simulink model "gm_rx_dma_test"  (R2024a)
settings: Solver=FixedStepDiscrete  StartTime=0.0  StopTime=2e-3  RelTol=1e-3  EnableMultiTasking=on
PreLoadFcn:
  | ldcr_hdl_init();
InitFcn:
  | ldcr_hdl_init();
model workspace (MAT data in the model file):
  socvcb = containers.Map
  socvcb.serialization.keys = {}
  socvcb.serialization.values = {}
  socvcb.serialization.uniformity = 0
  socvcb.serialization.keyType = 'double'
  socvcb.serialization.valueType = 'any'
libraries: dspsrcs4 x2, hdlsllib x2, dsphdlfiltering2 x1
Description:
  | libiioSDRPSP_filter_example
  | 
  | A simple example model to demonstrate the use of MATLAB I/O alongside
  | hardware/software co-design.
  | 
  | Implements AXI programmable gain and bypassable filters on the Tx and Rx
  | paths of the HDL DUT.
settings Model: SimulationMode=accelerator  ExtModeTrigDuration=100  Creator=mfornero  LastModifiedBy=versal
settings SolverCC: AlgebraicLoopSolver=TrustRegion  PositivePriorityOrder=on  MaxZcPerStep=1
settings DataIOCC: SaveOutput=off  ReturnWorkspaceOutputs=off  StateSaveName=tmp_raccel_xout  SignalLoggingName=tmp_raccel_logsout
settings OptimizationCC: BlockReduction=off  ConditionallyExecuteInputs=off  DefaultParameterBehavior=Inlined  EnhancedBackFolding=on  PassReuseOutputArgsAs=Individual arguments  ZeroExternalMemoryAtStartup=off  ZeroInternalMemoryAtStartup=off  EfficientMapNaN2IntZero=off  MaxStackSize=64  OptimizeBlockOrder=speed  DifferentSizesBufferReuse=on  OptimizationCustomize=off  EfficientTunableParamExpr=on
settings DebuggingCC: AlgebraicLoopMsg=error  InheritedTsInSrcMsg=none  SingleTaskRateTransMsg=error  ParameterTunabilityLossMsg=error  UnconnectedInputMsg=warning  UnconnectedOutputMsg=warning  UnconnectedLineMsg=warning  PregeneratedLibrarySubsystemCodeDiagnostic=none  StrictBusMsg=ErrorOnBusTreatedAsVector  SFUnexpectedBacktrackingDiag=warning  SFNoUnconditionalDefaultTransitionDiag=warning  SFExecutionAtInitializationDiag=none  ArithmeticOperatorsInVariantConditions=warning
settings HardwareCC: ProdBitPerPointer=32  ProdBitPerSizeT=32  ProdBitPerPtrDiffT=32  ProdLargestAtomicFloat=None  ProdIntDivRoundTo=Undefined  ProdEndianess=Unspecified  ProdWordSize=32  ProdHWDeviceType=ASIC/FPGA->ASIC/FPGA  TargetBitPerLong=64  TargetBitPerPointer=64  TargetBitPerSizeT=64  TargetBitPerPtrDiffT=64  TargetLongLongMode=on  TargetIntDivRoundTo=Zero  TargetEndianess=LittleEndian  TargetWordSize=64  TargetHWDeviceType=Custom Processor->MATLAB Host Computer  ProdEqTarget=off  HardwareBoardFeatureSet=SoCBlockset
settings ModelReferenceCC: EnableRefExpFcnMdlSchedulingChecks=on  ModelReferenceNumInstancesAllowed=Single
settings SFSimCC: SimUseLocalCustomCode=off  CustomCodeUndefinedFunction=UseInterfaceOnly
settings RTWCC: Description=Embedded Coder  SystemTargetFile=ert.tlc  HardwareBoard=Custom Hardware Board  TLCOptions="-aInlineSetEventsForThisBaseRateFcn=TLC_FALSE -aSuppressMultiTaskScheduler=TLC_FALSE  -aRateBasedStepFcn=0"  TemplateMakefile=ert_default_tmf  RTWVerbose=off  RTWUseLocalCustomCode=off  RTWUseSimCustomCode=on  GPUComputeCapability=3.5  DLArmComputeVersion=19.05
settings CodeAppCC: ForceParamTrailComments=on  IgnoreCustomStorageClasses=off  MaxIdLength=128  OperatorAnnotations=on  SimulinkDataObjDesc=on  SFDataObjDesc=on  MangleLength=10  InsertBlockDesc=on
settings ERTTargetCC: InlinedParameterPlacement=NonHierarchical
settings ConfigComp: CovMetricSettings=dw  CovSaveCumulativeToWorkspaceVar=on  CovSaveSingleToWorkspaceVar=on  CovExternalEMLEnable=off

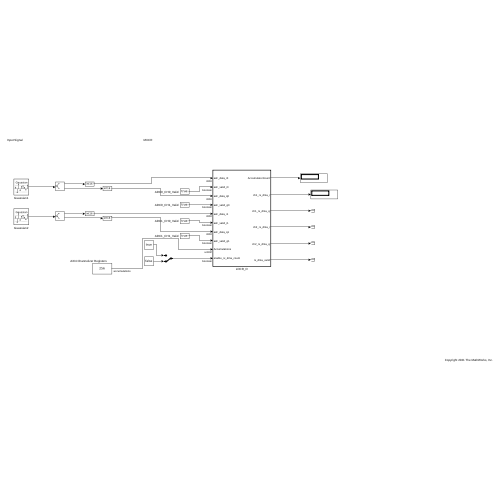
[thumbnail: Simulink's stored preview of the top-level diagram]
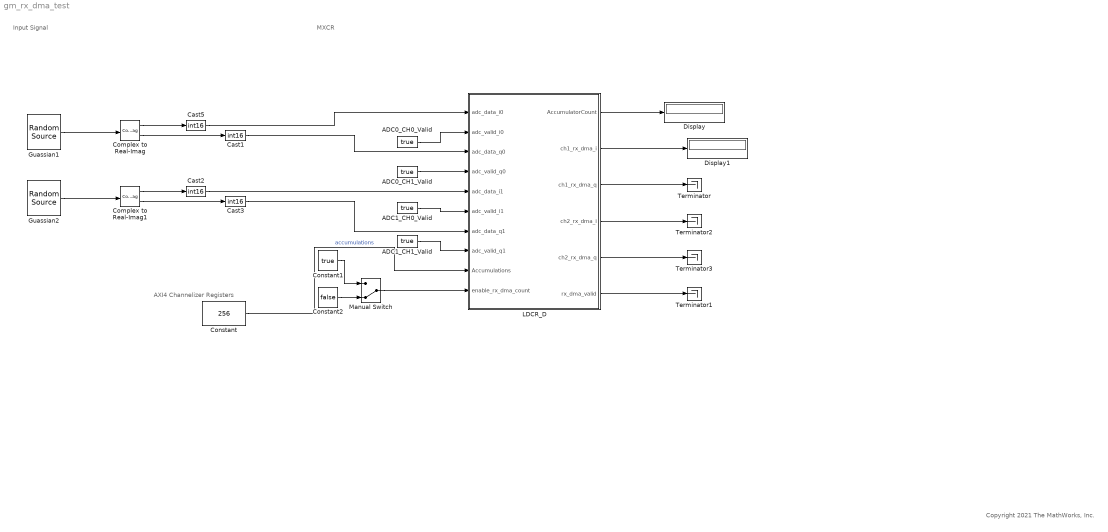
== system gm_rx_dma_test ==
  note: Input Signal
  note: MXCR
  note: Copyright 2021 The MathWorks, Inc.
  note: AXI4 Channelizer Registers
  ADC0_CH0_Valid : Constant  Value=true  SampleTime=-1
  ADC0_CH1_Valid : Constant  Value=true  SampleTime=-1
  ADC1_CH0_Valid : Constant  Value=true  SampleTime=-1
  ADC1_CH1_Valid : Constant  Value=true  SampleTime=-1
  Cast{1..3,5} (4 alike) : DataTypeConversion  OutDataTypeStr=int16  SaturateOnIntegerOverflow=off  RndMeth=Floor
  Complex to Real-Imag : ComplexToRealImag
  Complex to Real-Imag1 : ComplexToRealImag
  Constant : Constant  Value=256  OutDataTypeStr=uint32
  Constant1 : Constant  Value=true  SampleTime=-1
  Constant2 : Constant  Value=false  SampleTime=-1
  Display : Display
  Display1 : Display
  Guassian1 : dspsrcs4/Random Source  SrcType=Gaussian  MinVal=0  MaxVal=1  MeanVal=9  VarVal=24^2  RepMode=Specify seed  rawSeed=6547597  IsInherit=off  SampTime=Ts  SampFrame=1  OutComplex=Complex  DataType=single  SimulateUsing=Interpreted execution
  Guassian2 : dspsrcs4/Random Source  SrcType=Gaussian  MinVal=0  MaxVal=1  MeanVal=7  VarVal=24^2  RepMode=Specify seed  rawSeed=1324634  IsInherit=off  SampTime=Ts  SampFrame=1  OutComplex=Complex  DataType=single  SimulateUsing=Interpreted execution
  LDCR_D : Subsystem  TreatAsAtomicUnit=on
  Manual Switch : ManualSwitch  CurrentSetting=0
  Terminator{,1..3} (4 alike) : Terminator
  wires:
  Constant2/1 -> Manual Switch/2
  Constant1/1 -> Manual Switch/1
  LDCR_D/5(ch2_rx_dma_q) -> Terminator3/1
  LDCR_D/4(ch2_rx_dma_i) -> Terminator2/1
  LDCR_D/6(rx_dma_valid) -> Terminator1/1
  LDCR_D/3(ch1_rx_dma_q) -> Terminator/1
  Guassian2/1 -> Complex to Real-Imag1/1
  Guassian1/1 -> Complex to Real-Imag/1
  Cast3/1 -> LDCR_D/7(adc_data_q1)
  Cast2/1 -> LDCR_D/5(adc_data_i1)
  Cast1/1 -> LDCR_D/3(adc_data_q0)
  Cast5/1 -> LDCR_D/1(adc_data_i0)
  Complex to Real-Imag1/2 -> Cast3/1
  Complex to Real-Imag1/1 -> Cast2/1
  Complex to Real-Imag/2 -> Cast1/1
  Complex to Real-Imag/1 -> Cast5/1
  LDCR_D/1(AccumulatorCount) -> Display/1
  LDCR_D/2(ch1_rx_dma_i) -> Display1/1
  Manual Switch/1 -> LDCR_D/10(enable_rx_dma_count)
  ADC1_CH1_Valid/1 -> LDCR_D/8(adc_valid_q1)
  ADC1_CH0_Valid/1 -> LDCR_D/6(adc_valid_i1)
  ADC0_CH1_Valid/1 -> LDCR_D/4(adc_valid_q0)
  Constant/1 -> LDCR_D/9(Accumulations)  "accumulations"
  ADC0_CH0_Valid/1 -> LDCR_D/2(adc_valid_i0)

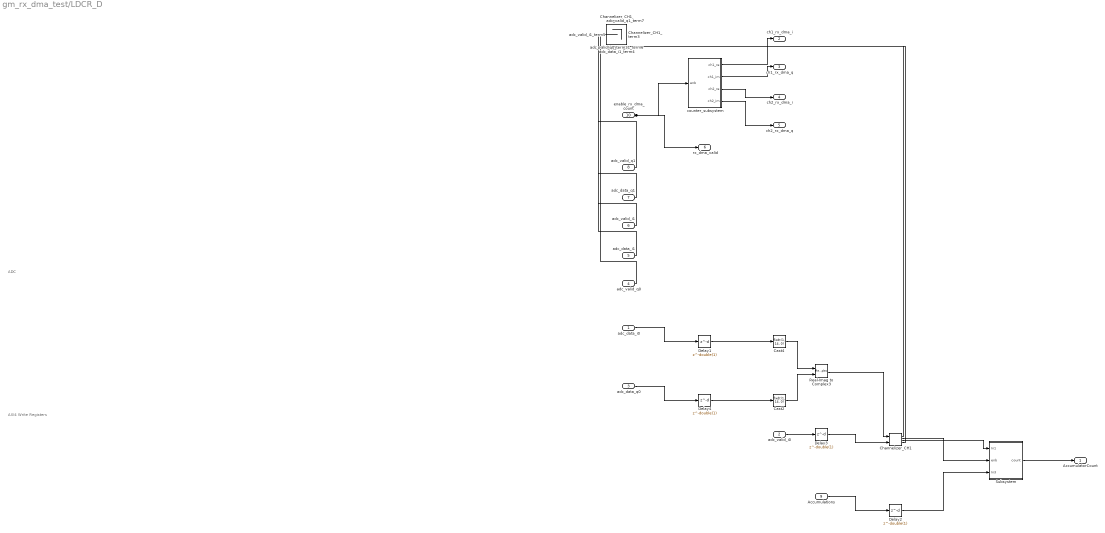
== system gm_rx_dma_test/LDCR_D ==
  note: ADC
  note: AXI4 Write Registers
  adc_data_i0 : Inport  OutDataTypeStr=int16  PortDimensions=1  SampleTime=3.25520833333333e-08
  adc_valid_i0 : Inport  Port=2  OutDataTypeStr=boolean  PortDimensions=1  SampleTime=3.25520833333333e-08
  adc_data_q0 : Inport  Port=3  OutDataTypeStr=int16  PortDimensions=1  SampleTime=3.25520833333333e-08
  adc_valid_q0 : Inport  Port=4  OutDataTypeStr=boolean  PortDimensions=1  SampleTime=3.25520833333333e-08
  adc_data_i1 : Inport  Port=5  OutDataTypeStr=int16  PortDimensions=1  SampleTime=3.25520833333333e-08
  adc_valid_i1 : Inport  Port=6  OutDataTypeStr=boolean  PortDimensions=1  SampleTime=3.25520833333333e-08
  adc_data_q1 : Inport  Port=7  OutDataTypeStr=int16  PortDimensions=1  SampleTime=3.25520833333333e-08
  adc_valid_q1 : Inport  Port=8  OutDataTypeStr=boolean  PortDimensions=1  SampleTime=3.25520833333333e-08
  Accumulations : Inport  Port=9  OutDataTypeStr=uint32  PortDimensions=1  SampleTime=3.25520833333333e-08
  enable_rx_dma_count : Inport  Port=10  OutDataTypeStr=boolean  PortDimensions=1  SampleTime=3.25520833333333e-08
  Cast2 : DataTypeConversion  OutDataTypeStr=fixdt(1, 14, 0)  SampleTime=3.25520833333333e-08  SaturateOnIntegerOverflow=off  RndMeth=Floor
  Cast4 : DataTypeConversion  OutDataTypeStr=fixdt(1, 14, 0)  SampleTime=3.25520833333333e-08  SaturateOnIntegerOverflow=off  RndMeth=Floor
  Channelizer_CH1 : dsphdlfiltering2/Channelizer  FilterCoefficients=pfb.coeffs.Numerator  FilterStructure=Direct form systolic  NumFrequencyBands=fftsize  ComplexMultiplication=Use 3 multipliers and 5 adders  Normalize=off  OutputSize=Same as input size  SimulateUsing=Code generation  roundingMode=Floor  overflowMode=off  CoefficientsDataTypeStr=Inherit: Same word length as input  FilterOutputDataTypeStr=Inherit: Same word length as input  ResetInputPort=off  StartOutputPort=on  EndOutputPort=on
  Channelizer_CH1_term0 : Terminator
  Channelizer_CH1_term3 : Terminator
  Delay{1..4} (4 alike) : Delay  DelayLength=double(1)  InitialCondition=0  SampleTime=3.25520833333333e-08
  Real-Imag to Complex3 : RealImagToComplex  ConstantPart="fi(0,1,14,0,\"hex\",\"0000\")"  SampleTime=3.25520833333333e-08
  Subsystem : Subsystem
  adc_data_i1_term4 : Terminator
  adc_data_q1_term6 : Terminator
  adc_valid_i1_term5 : Terminator
  adc_valid_q0_term3 : Terminator
  adc_valid_q1_term7 : Terminator
  counter_subsystem : Subsystem
  AccumulatorCount : Outport  SampleTime=3.25520833333333e-08  VectorParamsAs1DForOutWhenUnconnected=off
  ch1_rx_dma_i : Outport  Port=2  SampleTime=3.25520833333333e-08  VectorParamsAs1DForOutWhenUnconnected=off
  ch1_rx_dma_q : Outport  Port=3  SampleTime=3.25520833333333e-08
  ch2_rx_dma_i : Outport  Port=4  SampleTime=3.25520833333333e-08  VectorParamsAs1DForOutWhenUnconnected=off
  ch2_rx_dma_q : Outport  Port=5  SampleTime=3.25520833333333e-08
  rx_dma_valid : Outport  Port=6  SampleTime=3.25520833333333e-08
  wires:
  adc_data_i0/1 -> Delay1/1
  adc_valid_i0/1 -> Delay3/1
  adc_data_q0/1 -> Delay4/1
  adc_valid_q0/1 -> adc_valid_q0_term3/1
  adc_data_i1/1 -> adc_data_i1_term4/1
  adc_valid_i1/1 -> adc_valid_i1_term5/1
  adc_data_q1/1 -> adc_data_q1_term6/1
  adc_valid_q1/1 -> adc_valid_q1_term7/1
  Accumulations/1 -> Delay2/1
  enable_rx_dma_count/1 -> counter_subsystem/1(enb), rx_dma_valid/1
  Cast2/1 -> Real-Imag to Complex3/2
  Cast4/1 -> Real-Imag to Complex3/1
  Channelizer_CH1/1 -> Channelizer_CH1_term0/1
  Channelizer_CH1/2 -> Subsystem/2(enb)
  Channelizer_CH1/3 -> Subsystem/1(In1)
  Channelizer_CH1/4 -> Channelizer_CH1_term3/1
  Delay1/1 -> Cast4/1
  Delay2/1 -> Subsystem/3(In3)
  Delay3/1 -> Channelizer_CH1/2
  Delay4/1 -> Cast2/1
  Real-Imag to Complex3/1 -> Channelizer_CH1/1
  Subsystem/1(count) -> AccumulatorCount/1
  counter_subsystem/1(ch1_re) -> ch1_rx_dma_i/1
  counter_subsystem/2(ch1_im) -> ch1_rx_dma_q/1
  counter_subsystem/3(ch2_re) -> ch2_rx_dma_i/1
  counter_subsystem/4(ch2_im) -> ch2_rx_dma_q/1

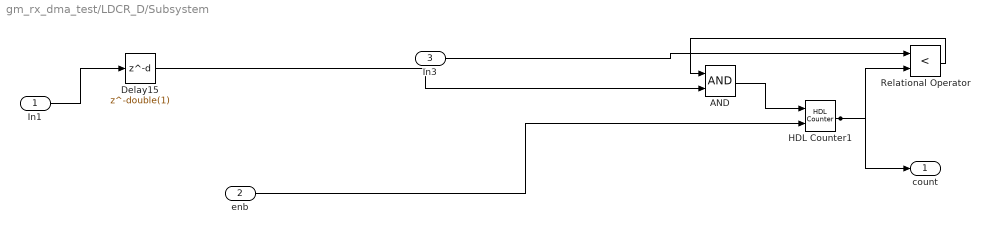
== system gm_rx_dma_test/LDCR_D/Subsystem ==
  In1 : Inport  OutDataTypeStr=boolean  PortDimensions=1  SampleTime=3.25520833333333e-08
  enb : Inport  Port=2  OutDataTypeStr=boolean  PortDimensions=1  SampleTime=3.25520833333333e-08
  In3 : Inport  Port=3  OutDataTypeStr=uint32  PortDimensions=1  SampleTime=3.25520833333333e-08
  AND : Logic  AllPortsSameDT=off  OutDataTypeStr=boolean  SampleTime=3.25520833333333e-08
  Delay15 : Delay  DelayLength=double(1)  InitialCondition=0  SampleTime=3.25520833333333e-08
  HDL Counter1 : hdlsllib/Sources/HDL Counter  CountType=Free running  CountInit=0  CountStep=1  CountMax=16  CountFromType=Initial value  CountFrom=0  CountResetPort=on  CountLoadPort=off  CountEnbPort=on  CountDirPort=off  CountHitOutputPort=off  CountDataType=Unsigned  CountWordLen=32  CountFracLen=0  CountSampTime=1
  Relational Operator : RelationalOperator  Operator=<  OutDataTypeStr=boolean  SampleTime=3.25520833333333e-08  InputSameDT=off
  count : Outport  SampleTime=3.25520833333333e-08
  wires:
  In1/1 -> Delay15/1
  enb/1 -> HDL Counter1/2
  In3/1 -> Relational Operator/1
  AND/1 -> HDL Counter1/1
  Delay15/1 -> AND/2
  HDL Counter1/1 -> Relational Operator/2, count/1
  Relational Operator/1 -> AND/1

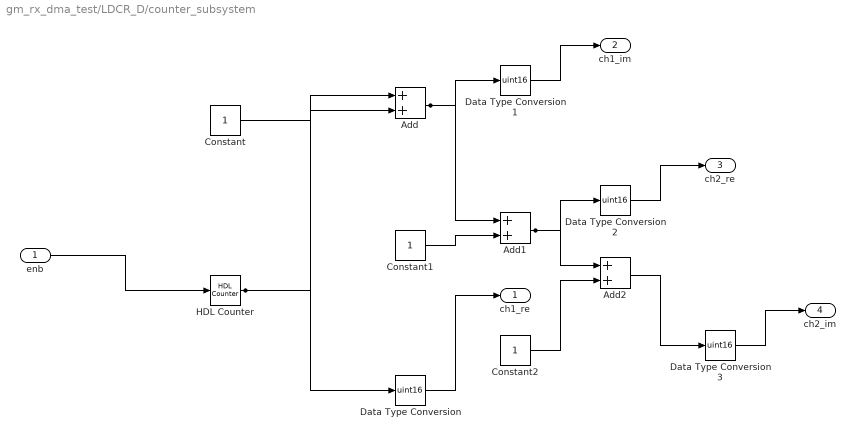
== system gm_rx_dma_test/LDCR_D/counter_subsystem ==
  enb : Inport  OutDataTypeStr=boolean  PortDimensions=1  SampleTime=3.25520833333333e-08
  Add : Sum  OutDataTypeStr=fixdt(0, 17, 0)  AccumDataTypeStr=fixdt(0, 17, 0)  SampleTime=3.25520833333333e-08
  Add1 : Sum  OutDataTypeStr=fixdt(0, 18, 0)  AccumDataTypeStr=fixdt(0, 18, 0)  SampleTime=3.25520833333333e-08
  Add2 : Sum  OutDataTypeStr=fixdt(0, 19, 0)  AccumDataTypeStr=fixdt(0, 19, 0)  SampleTime=3.25520833333333e-08
  Constant : Constant  OutDataTypeStr=uint16  SampleTime=3.25520833333333e-08
  Constant1 : Constant  OutDataTypeStr=uint16  SampleTime=3.25520833333333e-08
  Constant2 : Constant  OutDataTypeStr=uint16  SampleTime=3.25520833333333e-08
  Data Type Conversion{,1..3} (4 alike) : DataTypeConversion  OutDataTypeStr=uint16  SampleTime=3.25520833333333e-08  SaturateOnIntegerOverflow=off  RndMeth=Floor
  HDL Counter : hdlsllib/Sources/HDL Counter  CountType=Free running  CountInit=0  CountStep=4  CountMax=25  CountFromType=Initial value  CountFrom=0  CountResetPort=off  CountLoadPort=off  CountEnbPort=on  CountDirPort=off  CountHitOutputPort=off  CountDataType=Unsigned  CountWordLen=12  CountFracLen=0  CountSampTime=-1
  ch1_re : Outport  SampleTime=3.25520833333333e-08
  ch1_im : Outport  Port=2  SampleTime=3.25520833333333e-08
  ch2_re : Outport  Port=3  SampleTime=3.25520833333333e-08
  ch2_im : Outport  Port=4  SampleTime=3.25520833333333e-08
  wires:
  enb/1 -> HDL Counter/1
  Add/1 -> Data Type Conversion1/1, Add1/1
  Add1/1 -> Data Type Conversion2/1, Add2/1
  Add2/1 -> Data Type Conversion3/1
  Constant/1 -> Add/2
  Constant1/1 -> Add1/2
  Constant2/1 -> Add2/2
  Data Type Conversion/1 -> ch1_re/1
  Data Type Conversion1/1 -> ch1_im/1
  Data Type Conversion2/1 -> ch2_re/1
  Data Type Conversion3/1 -> ch2_im/1
  HDL Counter/1 -> Data Type Conversion/1, Add/1
